simulink model "RUNTHIS"  (R2021a)
settings: Solver=FixedStepAuto  StartTime=0.0  StopTime=10.0  RelTol=1e-3
settings Model: Creator=USER  LastModifiedBy=RICKY
settings SolverCC: AlgebraicLoopSolver=TrustRegion
settings DebuggingCC: SFMachineParentedDataDiag=warning

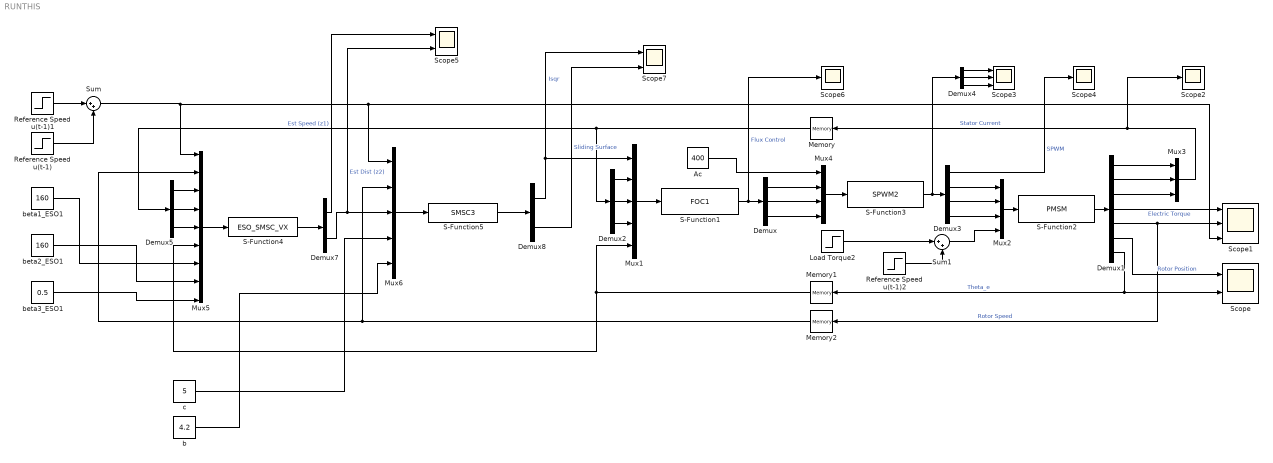
== system RUNTHIS ==
  Ac : Constant  Value=400
  Demux{,2,4..5} (4 alike) : Demux  Outputs=3
  Demux1 : Demux  Outputs=7
  Demux3 : Demux
  Demux7 : Demux  Outputs=2
  Demux8 : Demux  Outputs=2
  Load Torque2 : Step  Time=2  After=0  SampleTime=0
  Memory : Memory
  Memory1 : Memory
  Memory2 : Memory
  Mux1 : Mux  Inputs=5
  Mux2 : Mux
  Mux3 : Mux  Inputs=3
  Mux4 : Mux
  Mux5 : Mux  Inputs=9
  Mux6 : Mux  Inputs=5
  Reference Speed u(t-1) : Step  Time=5  After=-25  SampleTime=0
  Reference Speed u(t-1)1 : Step  After=50  SampleTime=0
  Reference Speed u(t-1)2 : Step  After=0  SampleTime=0
  S-Function1 : S-Function  FunctionName=FOC1  SFunctionDeploymentMode=off  EnableBusSupport=off
  S-Function2 : S-Function  FunctionName=PMSM  SFunctionDeploymentMode=off  EnableBusSupport=off
  S-Function3 : S-Function  FunctionName=SPWM2  SFunctionDeploymentMode=off  EnableBusSupport=off
  S-Function4 : S-Function  FunctionName=ESO_SMSC_VX  SFunctionDeploymentMode=off  EnableBusSupport=off
  S-Function5 : S-Function  FunctionName=SMSC3  SFunctionDeploymentMode=off  EnableBusSupport=off
  Scope : Scope  NumInputPorts=2
  Scope1 : Scope  NumInputPorts=3
  Scope2 : Scope
  Scope3 : Scope  NumInputPorts=3
  Scope4 : Scope
  Scope5 : Scope  NumInputPorts=2
  Scope6 : Scope
  Scope7 : Scope  NumInputPorts=2
  Sum : Sum  Inputs=|++
  Sum1 : Sum  Inputs=|++
  b : Constant  Value=4.2
  beta1_ESO1 : Constant  Value=160
  beta2_ESO1 : Constant  Value=160
  beta3_ESO1 : Constant  Value=0.5
  c : Constant  Value=5
  wires:
  Demux3/2 -> Mux2/1
  S-Function3/1 -> Demux4/1, Demux3/1
  Demux/2 -> Mux4/3
  Memory/1 -> Demux5/1, Demux2/1
  Demux4/2 -> Scope3/2
  Demux4/3 -> Scope3/3
  Mux4/1 -> S-Function3/1
  S-Function2/1 -> Demux1/1
  Demux3/3 -> Mux2/2
  Demux2/1 -> Mux1/2
  Demux/1 -> Mux4/2
  Demux1/6 -> Scope/1  "Rotor Position"
  Demux3/1 -> Scope4/1  "SPWM"
  Demux/3 -> Mux4/4
  Demux2/3 -> Mux1/4
  Demux1/7 -> Memory1/1, Scope/2  "Theta_e"
  Ac/1 -> Mux4/1
  Demux4/1 -> Scope3/1
  Mux1/1 -> S-Function1/1
  Demux1/4 -> Scope1/1  "Electric Torque"
  Demux1/5 -> Memory2/1, Scope1/2  "Rotor Speed"
  Mux3/1 -> Memory/1, Scope2/1  "Stator Current"
  Demux1/2 -> Mux3/2
  Demux2/2 -> Mux1/3
  Demux3/4 -> Mux2/3
  Demux1/1 -> Mux3/1
  Demux1/3 -> Mux3/3
  Mux2/1 -> S-Function2/1
  S-Function1/1 -> Scope6/1, Demux/1  "Flux Control"
  Mux5/1 -> S-Function4/1
  S-Function4/1 -> Demux7/1
  Mux6/1 -> S-Function5/1
  S-Function5/1 -> Demux8/1
  Demux8/1 -> Scope7/1, Mux1/1  "Isqr"
  Memory2/1 -> Mux6/2, Mux5/2
  c/1 -> Mux6/4
  b/1 -> Mux6/5
  beta3_ESO1/1 -> Mux5/9
  beta2_ESO1/1 -> Mux5/8
  beta1_ESO1/1 -> Mux5/7
  Demux5/1 -> Mux5/3
  Demux5/3 -> Mux5/5
  Demux5/2 -> Mux5/4
  Memory1/1 -> Mux5/6, Mux1/5
  Demux7/2 -> Scope5/2, Mux6/3  "Est Dist (z2)"
  Demux7/1 -> Scope5/1  "Est Speed (z1)"
  Demux8/2 -> Scope7/2  "Sliding Surface"
  Sum/1 -> Mux6/1, Scope1/3, Mux5/1
  Reference Speed u(t-1)1/1 -> Sum/1
  Reference Speed u(t-1)/1 -> Sum/2
  Sum1/1 -> Mux2/4
  Load Torque2/1 -> Sum1/1
  Reference Speed u(t-1)2/1 -> Sum1/2
